simulink model "distmodelR2019a"  (R2019a)
settings: Solver=FixedStepAuto  StartTime=0.0  StopTime=t_sim  FixedStep=TimeStep  RelTol=1e-3
values from neighbouring files (symbols this model uses):
  alt = 300    [main_disturbances.m]    (also in simple_propagator.m)
  D = [x_th-x_cog;y_th-y_cog;z_th-z_cog]/1e3    [momentumstorage.m]
  inc = rad2deg(inc)    [main_disturbances.m]    (also in simple_propagator.m)
  nu = rad2deg(nu)    [main_disturbances.m]    (also in simple_propagator.m)
  RAAN = rad2deg(RAAN)    [main_disturbances.m]    (also in simple_propagator.m)
  w = find(volume(:,y,z) == 1)    [calc_torque_v1.m]    (also in main_disturbances.m = rad2deg(w); simple_propagator.m = rad2deg(w))
undefined symbols (not defined in the file or in its folder): date, ecc, km, LOAS, s, sat
libraries: vrlib x4, dspmathops x4, sharedtransform x3, simulink_extras x2, aerolibutil x2, aerolibatmos2 x1, dspindex x1, aerolibcelestial x1, sharedutil x1
settings Model: Creator=colpari  LastModifiedBy=colpari

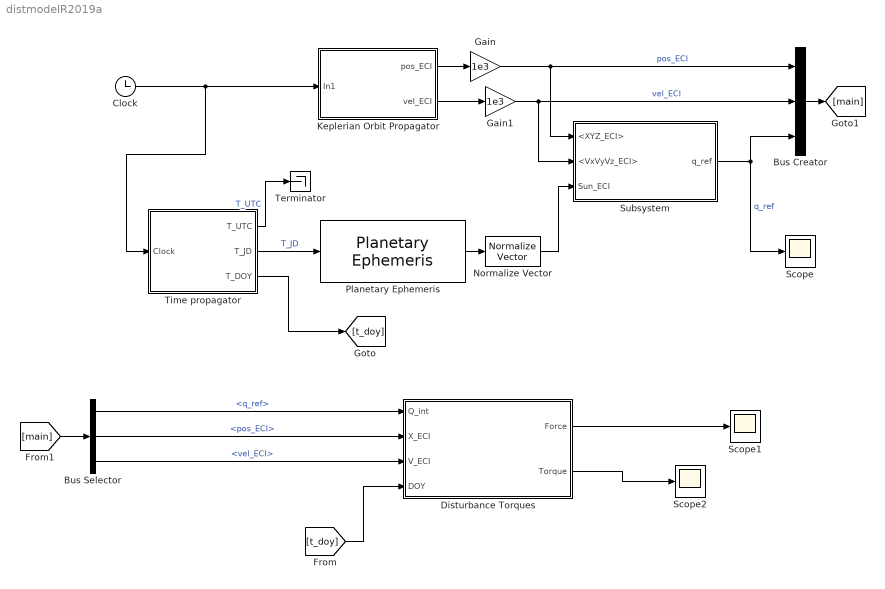
== system distmodelR2019a ==
  Bus Creator : BusCreator  Inputs=3
  Bus Selector : BusSelector  OutputSignals=q_ref,pos_ECI,vel_ECI
  Clock : Clock
  "Disturbance Torques " : Subsystem
  Gain : Gain  Gain=1e3
  Gain1 : Gain  Gain=1e3
  Keplerian Orbit Propagator : Subsystem
  Normalize Vector : vrlib/Utilities/Normalize Vector  maxzero=0
  Planetary Ephemeris : aerolibcelestial/Planetary Ephemeris  kmflag=km,km/s  epochflag=Julian date  de=DE405  nCenter=Earth  nTarget=Sun  errorflag=Error  velflag=off
      settings: SourceProductBaseCode=AE
  Scope : Scope
  Scope1 : Scope
  Scope2 : Scope
  Subsystem : Subsystem
  Terminator : Terminator
  Time propagator : Subsystem
  wires:
  [t_doy] -> "Disturbance Torques "/4(DOY)
  "Disturbance Torques "/2("Torque ") -> Scope2/1
  "Disturbance Torques "/1(Force) -> Scope1/1
  Bus Selector/3 -> "Disturbance Torques "/3(V_ECI)  "<vel_ECI>"
  Bus Selector/2 -> "Disturbance Torques "/2(X_ECI)  "<pos_ECI>"
  Bus Selector/1 -> "Disturbance Torques "/1("Q_int ")  "<q_ref>"
  Clock/1 -> Keplerian Orbit Propagator/1(In1), Time propagator/1(Clock)
  Keplerian Orbit Propagator/1(pos_ECI) -> Gain/1
  Keplerian Orbit Propagator/2(vel_ECI) -> Gain1/1
  Planetary Ephemeris/1 -> Normalize Vector/1
  Normalize Vector/1 -> Subsystem/3(Sun_ECI)
  Time propagator/2(T_JD) -> Planetary Ephemeris/1  "T_JD"
  Subsystem/1(q_ref) -> Bus Creator/3, Scope/1  "q_ref"
  Time propagator/3(T_DOY) -> [t_doy]
  Bus Creator/1 -> [main]
  Time propagator/1(T_UTC) -> Terminator/1  "T_UTC"
  [main] -> Bus Selector/1
  Gain/1 -> Subsystem/1(<XYZ_ECI>), Bus Creator/1  "pos_ECI"
  Gain1/1 -> Subsystem/2(<VxVyVz_ECI>), Bus Creator/2  "vel_ECI"

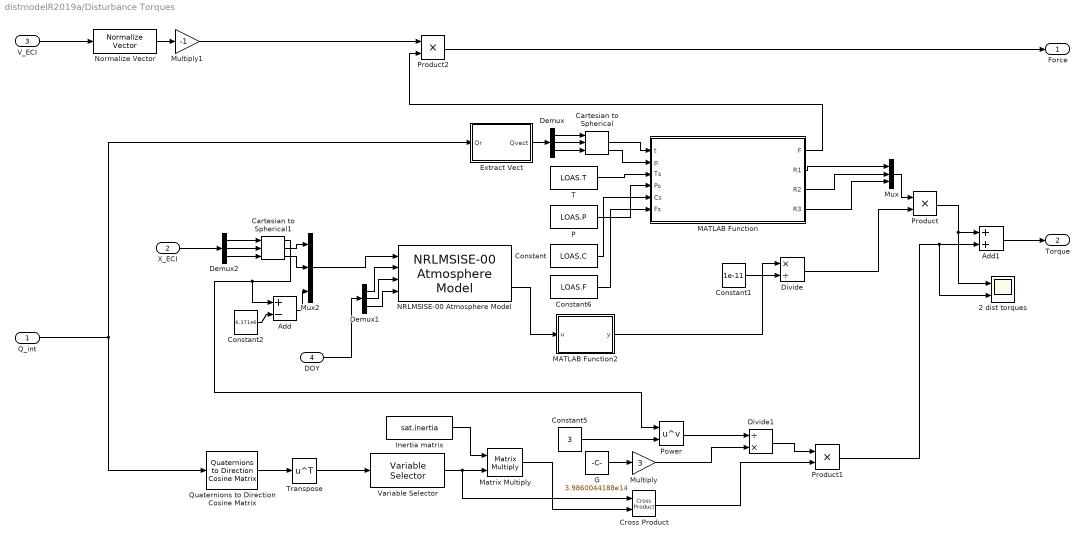
== system distmodelR2019a/Disturbance Torques  ==
  "Q_int " : Inport
  X_ECI : Inport  Port=2
  V_ECI : Inport  Port=3
  DOY : Inport  Port=4
  2 dist torques : Scope  NumInputPorts=2
  Add : Sum  Inputs=+-
  Add1 : Sum
  Cartesian to Spherical : simulink_extras/Transformations/Cartesian to Spherical
      settings: SourceProductBaseCode=SL
  Cartesian to Spherical1 : simulink_extras/Transformations/Cartesian to Spherical
      settings: SourceProductBaseCode=SL
  Constant : Constant  Value=LOAS.C
  Constant1 : Constant  Value=1e-11
  Constant2 : Constant  Value=6.371e6
  Constant5 : Constant  Value=3
  Constant6 : Constant  Value=LOAS.F
  Cross Product : vrlib/Utilities/Cross Product
  Demux : Demux  Outputs=3
  Demux1 : Demux  Outputs=3
  Demux2 : Demux  Outputs=3
  Divide : Product  Inputs=*/
  Divide1 : Product  Inputs=/*
  Extract Vect : Subsystem
  G : Constant  Value=3.9860044188e14
  Inertia matrix : Constant  Value=sat.inertia
  MATLAB Function : MATLAB Function  TreatAsAtomicUnit=on
  MATLAB Function2 : MATLAB Function  TreatAsAtomicUnit=on
  Matrix Multiply : Product  Multiplication=Matrix(*)
  Multiply : Gain  Gain=3
  Multiply1 : Gain  Gain=-1
  Mux : Mux  Inputs=3
  Mux2 : Mux  Inputs=3
  NRLMSISE-00 Atmosphere Model : aerolibatmos2/NRLMSISE-00 Atmosphere Model  units=Metric (MKS)  lst_input=off  flux_ap_input=off  flags_input=Internal  flags=ones(1,23)  oxygen_in=on  action=Warning
      settings: SourceProductBaseCode=AE
  Normalize Vector : vrlib/Utilities/Normalize Vector  maxzero=0
  "P " : Constant  Value=LOAS.P
  Power : Math  Operator=pow  SaturateOnIntegerOverflow=on
  Product : Product
  Product1 : Product
  Product2 : Product
  Quaternions to Direction Cosine Matrix : sharedtransform/Quaternions to  Direction Cosine Matrix  aMode=aMode
      settings: SourceProductBaseCode=AE,PW,MT,UV,VE,VP
  "T " : Constant  Value=LOAS.T
  Transpose : Math  Operator=transpose  SaturateOnIntegerOverflow=on
  Variable Selector : dspindex/Variable Selector  NumInputs=1  rowsOrCols=Columns  IdxMode=Fixed  Elements=[3]  ZerOneIdxMode=One-based  errmode=Clip Index  FillMode=on  FillValues=0
  Force : Outport
  "Torque " : Outport  Port=2
  wires:
  Constant/1 -> MATLAB Function/5(Cs)
  Extract Vect/1(Qvect) -> Demux/1
  Constant5/1 -> Power/2
  "T "/1 -> MATLAB Function/3(Ts)
  Quaternions to Direction Cosine Matrix/1 -> Transpose/1
  MATLAB Function/3(R2) -> Mux/2
  MATLAB Function/1(F) -> Product2/2
  Add/1 -> Mux2/3
  V_ECI/1 -> Normalize Vector/1
  Multiply1/1 -> Product2/1
  Cross Product/1 -> Product1/2
  Product1/1 -> 2 dist torques/2, Add1/2
  Multiply/1 -> Divide1/2
  Demux1/1 -> NRLMSISE-00 Atmosphere Model/2
  Divide1/1 -> Product1/1
  Matrix Multiply/1 -> Cross Product/2
  Demux2/3 -> Cartesian to Spherical1/3
  Demux2/1 -> Cartesian to Spherical1/1
  G/1 -> Multiply/1
  Cartesian to Spherical1/1 -> Add/1, Power/1
  Demux/1 -> Cartesian to Spherical/1
  Cartesian to Spherical/2 -> MATLAB Function/1(t)
  Inertia matrix/1 -> Matrix Multiply/1
  Variable Selector/1 -> Cross Product/1, Matrix Multiply/2
  Transpose/1 -> Variable Selector/1
  Product/1 -> 2 dist torques/1, Add1/1
  Divide/1 -> Product/2
  Constant2/1 -> Add/2
  Demux2/2 -> Cartesian to Spherical1/2
  Demux1/2 -> NRLMSISE-00 Atmosphere Model/3
  Cartesian to Spherical1/3 -> Mux2/2
  NRLMSISE-00 Atmosphere Model/2 -> MATLAB Function2/1(u)
  Normalize Vector/1 -> Multiply1/1
  MATLAB Function2/1(y) -> Divide/1
  Demux1/3 -> NRLMSISE-00 Atmosphere Model/4
  Cartesian to Spherical1/2 -> Mux2/1
  DOY/1 -> Demux1/1
  MATLAB Function/4(R3) -> Mux/3
  Constant1/1 -> Divide/2
  "Q_int "/1 -> Quaternions to Direction Cosine Matrix/1, Extract Vect/1(Qr)
  Demux/3 -> Cartesian to Spherical/3
  Demux/2 -> Cartesian to Spherical/2
  Constant6/1 -> MATLAB Function/6(Fs)
  Add1/1 -> "Torque "/1
  Product2/1 -> Force/1
  MATLAB Function/2(R1) -> Mux/1
  Mux2/1 -> NRLMSISE-00 Atmosphere Model/1
  X_ECI/1 -> Demux2/1
  Mux/1 -> Product/1
  Power/1 -> Divide1/1
  Cartesian to Spherical/3 -> MATLAB Function/2(p)
  "P "/1 -> MATLAB Function/4(Ps)

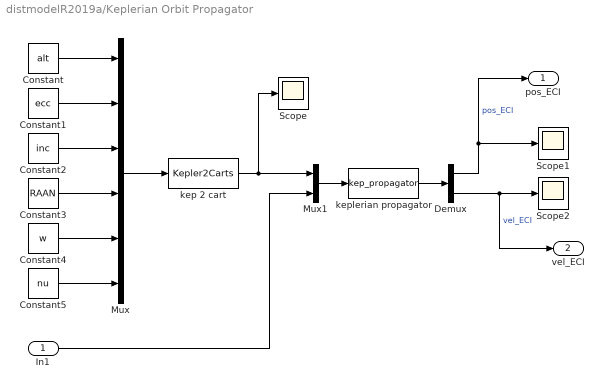
== system distmodelR2019a/Keplerian Orbit Propagator ==
  In1 : Inport
  Constant : Constant  Value=alt
  Constant1 : Constant  Value=ecc
  Constant2 : Constant  Value=inc
  Constant3 : Constant  Value=RAAN
  Constant4 : Constant  Value=w
  Constant5 : Constant  Value=nu
  Demux : Demux  Outputs=2
  Mux : Mux  Inputs=6
  Mux1 : Mux  Inputs=2
  Scope : Scope
  Scope1 : Scope
  Scope2 : Scope
  kep 2 cart : MATLABFcn  MATLABFcn=Kepler2Carts
  keplerian propagator : MATLABFcn  MATLABFcn=kep_propagator
  pos_ECI : Outport
  vel_ECI : Outport  Port=2
  wires:
  Mux/1 -> kep 2 cart/1
  Constant5/1 -> Mux/6
  Constant2/1 -> Mux/3
  kep 2 cart/1 -> Mux1/1, Scope/1
  Demux/2 -> vel_ECI/1, Scope2/1  "vel_ECI"
  Constant3/1 -> Mux/4
  Demux/1 -> pos_ECI/1, Scope1/1  "pos_ECI"
  Constant4/1 -> Mux/5
  keplerian propagator/1 -> Demux/1
  Mux1/1 -> keplerian propagator/1
  Constant/1 -> Mux/1
  Constant1/1 -> Mux/2
  In1/1 -> Mux1/2

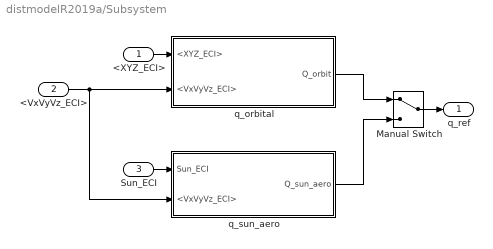
== system distmodelR2019a/Subsystem ==
  <XYZ_ECI> : Inport
  <VxVyVz_ECI> : Inport  Port=2
  Sun_ECI : Inport  Port=3
  Manual Switch : ManualSwitch
  q_orbital : Subsystem
  q_sun_aero : Subsystem
  q_ref : Outport
  wires:
  q_sun_aero/1(Q_sun_aero) -> Manual Switch/2
  <VxVyVz_ECI>/1 -> q_sun_aero/2(<VxVyVz_ECI>), q_orbital/2(<VxVyVz_ECI>)
  q_orbital/1(Q_orbit) -> Manual Switch/1
  Sun_ECI/1 -> q_sun_aero/1(Sun_ECI)
  Manual Switch/1 -> q_ref/1
  <XYZ_ECI>/1 -> q_orbital/1(<XYZ_ECI>)

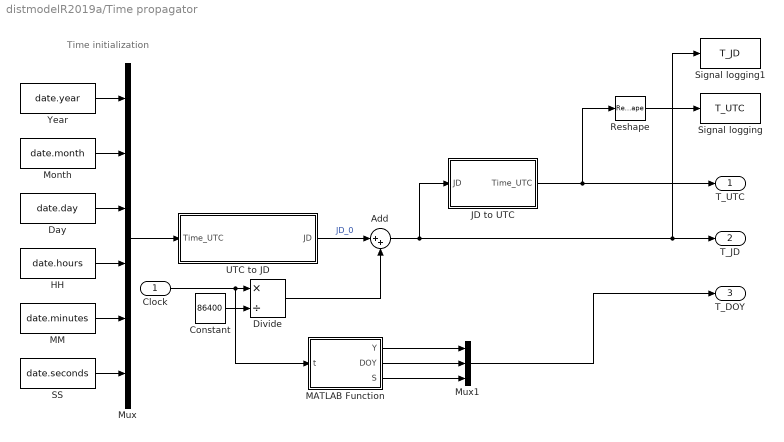
== system distmodelR2019a/Time propagator ==
  note: Time initialization
  Clock : Inport
  Add : Sum  Inputs=|++
  Constant : Constant  Value=86400
  Day : Constant  Value=date.day
  Divide : Product  Inputs=*/
  HH : Constant  Value=date.hours
  JD to UTC : MATLAB Function  TreatAsAtomicUnit=on
  MATLAB Function : MATLAB Function  TreatAsAtomicUnit=on
  MM : Constant  Value=date.minutes
  Month : Constant  Value=date.month
  Mux : Mux  Inputs=6
  Mux1 : Mux  Inputs=3
  Reshape : Reshape
  SS : Constant  Value=date.seconds
  Signal logging : ToWorkspace  VariableName=T_UTC  SaveFormat=Timeseries  SampleTime=1
      settings: Save2DSignal=2-D array (concatenate along first dimension)
  Signal logging1 : ToWorkspace  VariableName=T_JD  SaveFormat=Timeseries  SampleTime=1
      settings: Save2DSignal=2-D array (concatenate along first dimension)
  UTC to JD : MATLAB Function  TreatAsAtomicUnit=on
  Year : Constant  Value=date.year
  T_UTC : Outport  VectorParamsAs1DForOutWhenUnconnected=off
  T_JD : Outport  Port=2  VectorParamsAs1DForOutWhenUnconnected=off
  T_DOY : Outport  Port=3
  wires:
  UTC to JD/1(JD) -> Add/1  "JD_0"
  Clock/1 -> MATLAB Function/1(t), Divide/1
  Constant/1 -> Divide/2
  JD to UTC/1(Time_UTC) -> T_UTC/1, Reshape/1
  Divide/1 -> Add/2
  Mux/1 -> UTC to JD/1(Time_UTC)
  Day/1 -> Mux/3
  Month/1 -> Mux/2
  Year/1 -> Mux/1
  HH/1 -> Mux/4
  MM/1 -> Mux/5
  SS/1 -> Mux/6
  Reshape/1 -> Signal logging/1
  Add/1 -> Signal logging1/1, T_JD/1, JD to UTC/1(JD)
  MATLAB Function/1(Y) -> Mux1/1
  MATLAB Function/2(DOY) -> Mux1/2
  MATLAB Function/3(S) -> Mux1/3
  Mux1/1 -> T_DOY/1

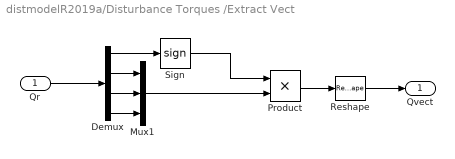
== system distmodelR2019a/Disturbance Torques /Extract Vect ==
  Qr : Inport
  Demux : Demux
  Mux1 : Mux  Inputs=3
  Product : Product
  Reshape : Reshape  OutputDimensionality=Column vector (2-D)
  Sign : Signum
  Qvect : Outport  VectorParamsAs1DForOutWhenUnconnected=off
  wires:
  Demux/2 -> Mux1/1
  Demux/4 -> Mux1/3
  Demux/3 -> Mux1/2
  Demux/1 -> Sign/1
  Qr/1 -> Demux/1
  Mux1/1 -> Product/2
  Product/1 -> Reshape/1
  Sign/1 -> Product/1
  Reshape/1 -> Qvect/1

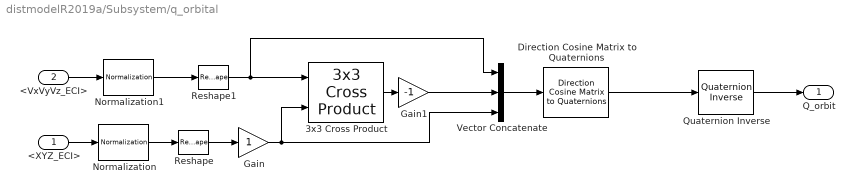
== system distmodelR2019a/Subsystem/q_orbital ==
  <XYZ_ECI> : Inport
  <VxVyVz_ECI> : Inport  Port=2
  3x3 Cross Product : sharedutil/3x3 Cross Product  aMode=aMode
      settings: SourceProductBaseCode=AE,PW,MT,UV,VE,VP
  Direction Cosine Matrix to Quaternions : sharedtransform/Direction Cosine Matrix  to Quaternions  aMode=0  action=None  tolerance=eps(2)
      settings: SourceProductBaseCode=AE,PW,MT,UV,VE,VP
  Gain : Gain
  Gain1 : Gain  Gain=-1
  Normalization : dspmathops/Normalization  NormType=2-norm  Bias=1e-10  NormOver=Each column  Dimension=1  roundingMode=Floor  overflowMode=off  accumDataTypeStr=Inherit: Same as product output  accumLastDataTypeStr=Inherit: Same as product output  outputDataTypeStr=Inherit: Same as product output  outputMin=[]  outputMax=[]  outputLastDataTypeStr=Inherit: Same as product output
  Normalization1 : dspmathops/Normalization  NormType=2-norm  Bias=1e-10  NormOver=Each column  Dimension=1  roundingMode=Floor  overflowMode=off  accumDataTypeStr=Inherit: Same as product output  accumLastDataTypeStr=Inherit: Same as product output  outputDataTypeStr=Inherit: Same as product output  outputMin=[]  outputMax=[]  outputLastDataTypeStr=Inherit: Same as product output
  Quaternion Inverse : aerolibutil/Quaternion Inverse
  Reshape : Reshape  OutputDimensionality=Column vector (2-D)
  Reshape1 : Reshape  OutputDimensionality=Column vector (2-D)
  Vector Concatenate : Concatenate  NumInputs=3  Mode=Multidimensional array  ConcatenateDimension=2
  Q_orbit : Outport  VectorParamsAs1DForOutWhenUnconnected=off
  wires:
  Normalization/1 -> Reshape/1
  Normalization1/1 -> Reshape1/1
  <VxVyVz_ECI>/1 -> Normalization1/1
  Reshape1/1 -> 3x3 Cross Product/1, Vector Concatenate/1
  <XYZ_ECI>/1 -> Normalization/1
  Reshape/1 -> Gain/1
  Gain/1 -> 3x3 Cross Product/2, Vector Concatenate/3
  Direction Cosine Matrix to Quaternions/1 -> Quaternion Inverse/1
  3x3 Cross Product/1 -> Gain1/1
  Gain1/1 -> Vector Concatenate/2
  Quaternion Inverse/1 -> Q_orbit/1
  Vector Concatenate/1 -> Direction Cosine Matrix to Quaternions/1

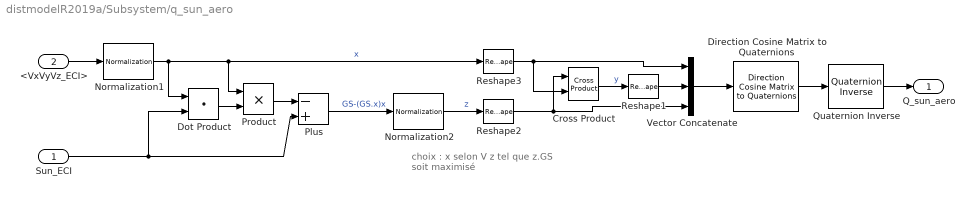
== system distmodelR2019a/Subsystem/q_sun_aero ==
  note: choix :
      | x selon V
      | z tel que z.GS soit maximisé
  Sun_ECI : Inport
  <VxVyVz_ECI> : Inport  Port=2
  Cross Product : vrlib/Utilities/Cross Product
  Direction Cosine Matrix to Quaternions : sharedtransform/Direction Cosine Matrix  to Quaternions  aMode=0  action=None  tolerance=eps(2)
      settings: SourceProductBaseCode=AE,PW,MT,UV,VE,VP
  Dot Product : DotProduct  InputSameDT=on  OutDataTypeStr=Inherit: Inherit via internal rule
  Normalization1 : dspmathops/Normalization  NormType=2-norm  Bias=1e-10  NormOver=Each column  Dimension=1  roundingMode=Floor  overflowMode=off  accumDataTypeStr=Inherit: Same as product output  accumLastDataTypeStr=Inherit: Same as product output  outputDataTypeStr=Inherit: Same as product output  outputMin=[]  outputMax=[]  outputLastDataTypeStr=Inherit: Same as product output
  Normalization2 : dspmathops/Normalization  NormType=2-norm  Bias=1e-10  NormOver=Each column  Dimension=1  roundingMode=Floor  overflowMode=off  accumDataTypeStr=Inherit: Same as product output  accumLastDataTypeStr=Inherit: Same as product output  outputDataTypeStr=Inherit: Same as product output  outputMin=[]  outputMax=[]  outputLastDataTypeStr=Inherit: Same as product output
  Plus : Sum  Inputs=-+
  Product : Product
  Quaternion Inverse : aerolibutil/Quaternion Inverse
  Reshape1 : Reshape  OutputDimensionality=Column vector (2-D)
  Reshape2 : Reshape  OutputDimensionality=Column vector (2-D)
  Reshape3 : Reshape  OutputDimensionality=Column vector (2-D)
  Vector Concatenate : Concatenate  NumInputs=3  Mode=Multidimensional array  ConcatenateDimension=2
  Q_sun_aero : Outport  VectorParamsAs1DForOutWhenUnconnected=off
  wires:
  Quaternion Inverse/1 -> Q_sun_aero/1
  Reshape2/1 -> Vector Concatenate/3, Cross Product/1
  Reshape3/1 -> Vector Concatenate/1, Cross Product/2
  Product/1 -> Plus/1
  Dot Product/1 -> Product/2
  Cross Product/1 -> Reshape1/1  "y"
  Normalization2/1 -> Reshape2/1  "z"
  Plus/1 -> Normalization2/1  "GS-(GS.x)x"
  Sun_ECI/1 -> Dot Product/2, Plus/2
  Vector Concatenate/1 -> Direction Cosine Matrix to Quaternions/1
  Direction Cosine Matrix to Quaternions/1 -> Quaternion Inverse/1
  Normalization1/1 -> Dot Product/1, Product/1, Reshape3/1  "x"
  <VxVyVz_ECI>/1 -> Normalization1/1
  Reshape1/1 -> Vector Concatenate/2

== matlab function distmodelR2019a/Disturbance Torques /MATLAB Function ==
  data: F output; t input; R1 output; p input; Ts input; Ps input; Cs input; Fs input; R2 output; R3 output
function [F, R1, R2, R3]   = interpol(t,p,Ts, Ps, Cs, Fs)
    norm1 = 0 ;
    sum1 = 0;
    norm2 = 0;
    sum2= 0;
    norm3 = 0;
    sum3 = 0;
    norm4 = 0;
    sum4 = 0;
    s=0.1;
    for i=1:500
        t2 = Ts(i,1);
        p2 = Ps(i,1);
        c1 = Cs(i,1);
        c2 = Cs(i,2);
        c3 = Cs(i,3);
        f1 = Fs(i,1);
        dist = distance_on_sphere(t,p,t2,p2);
        if dist<1e-10
            R1 = c1;
            R2 = c2;
            R3 = c3;
            F = f1;
        end  
        coef = (1/dist)^s;
        sum1 = sum1 + coef*c1;
        norm1 = norm1+coef;
        R1 = sum1/norm1;
        sum2 = sum2 + coef*c2;
        norm2 = norm2+coef;
        R2 = sum2/norm2;
        sum3 = sum3 + coef*c3;
        norm3 = norm3+coef;
        R3 = sum3/norm3;
        sum4 = sum4 + coef*f1;
        norm4 = norm4+coef;
        F = sum4/norm4;
    end
end

== matlab function distmodelR2019a/Disturbance Torques /MATLAB Function2 ==
  data: u input; y output
function y = fcn(u)
y = u(6);

== matlab function distmodelR2019a/Time propagator/UTC to JD ==
  data: Time_UTC input; JD output
function JD = fcn(Time_UTC)

% JD = juliandate(Time_UTC);
JD = Dt2jD(Time_UTC);

== matlab function distmodelR2019a/Time propagator/JD to UTC ==
  data: JD input; Time_UTC output
function Time_UTC = fcn(JD)
    coder.extrinsic('datetime','datevec');
    Time_UTC = [0,0,0,0,0,0];
Time_UTC =  datevec(datetime(JD,'convertfrom','juliandate'));

== matlab function distmodelR2019a/Time propagator/MATLAB Function ==
  data: t input; Y output; DOY output; S output
function [Y, DOY, S] = DOY(t)
Y = 2022 + fix(t/31557600);
DOY = 1+fix((t-floor(t/31557600)*31557600)/86400);
S = t - fix(t/31557600)*31557600 - (DOY-1)*86400;
